simulink model "sfcndemo_fcncallgen"  (Simulink 7.6)
settings: Solver=FixedStepDiscrete  StartTime=0.0  StopTime=10  MaxStep=0.0001  RelTol=1e-3
libraries: simulink x1
Description:
  | Function-call Generator Using C-MEX S-function
settings Model: Creator=The MathWorks Inc.  ExtModeTrigMode=oneshot  ExtModeArmWhenConnect=off  ExtModeAutoUpdateStatusClock=off
settings DataIOCC: LimitDataPoints=off
settings OptimizationCC: BlockReduction=off  BooleanDataType=off  InlineInvariantSignals=on  InitFltsAndDblsToZero=on
settings DebuggingCC: SaveWithParameterizedLinksMsg=none  SignalResolutionControl=TryResolveAllWithWarning  SolverPrmCheckMsg=none  MultiTaskDSMMsg=warning  MultiTaskCondExecSysMsg=none
settings HardwareCC: TargetUnknown=on
settings RTWCC: IncludeERTFirstTime=on
settings CodeAppCC: CustomSymbolStrFcn=$F$N$M
settings GRTTargetCC: TargetFcnLib=ansi_tfl_tmw.mat

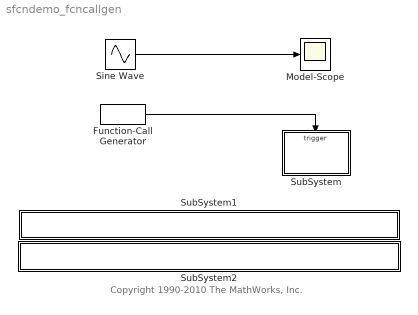
== system sfcndemo_fcncallgen ==
  note: Copyright 1990-2010 The MathWorks, Inc.
  Function-Call Generator : simulink/Ports & Subsystems/Function-Call Generator  sample_time=1  numberOfIterations=1
  Model-Scope : Scope
      settings: TimeRange=10
  Sine Wave : Sin  Amplitude=5  SampleTime=0.01
  SubSystem : Subsystem  TreatAsAtomicUnit=on
  SubSystem1 : Subsystem
      settings: OpenFcn=edit(fullfile(matlabroot,'toolbox','simulink','simdemos','simfeatures','sldemo_sfun_fcncallgen.c'))
      mask Display: disp('matlabroot\toolbox\simulink\simdemos\simfeatures\sldemo_sfun_fcncallgen.c');
  SubSystem2 : Subsystem
      settings: OpenFcn=edit(fullfile(matlabroot,'toolbox','simulink','simdemos','simfeatures','sldemo_sfun_fcncallgen.tlc'))
      mask Display: disp('matlabroot\toolbox\simulink\simdemos\simfeatures\sldemo_sfun_fcncallgen.tlc');
  wires:
  Sine Wave/1 -> Model-Scope/1
  Function-Call Generator/1 -> SubSystem/Trigger

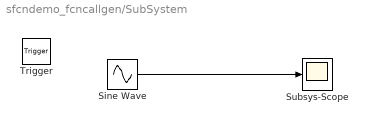
== system sfcndemo_fcncallgen/SubSystem ==
  Trigger : TriggerPort  TriggerType=function-call
  Sine Wave : Sin
  Subsys-Scope : Scope
      settings: TimeRange=10  YMin=-1  YMax=1
  wires:
  Sine Wave/1 -> Subsys-Scope/1

== system sfcndemo_fcncallgen/SubSystem1 ==

== system sfcndemo_fcncallgen/SubSystem2 ==
